simulink model "untitled"  (Simulink 7.9)
settings: Solver=ode45  StartTime=0.0  StopTime=10.0  RelTol=1e-3
settings Model: Creator=Administrator  LastModifiedBy=Administrator

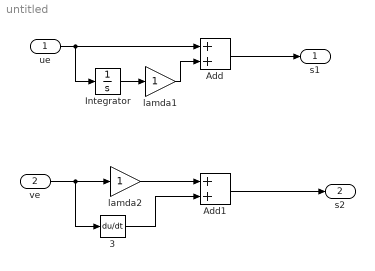
== system untitled ==
  ue : Inport
  ve : Inport  Port=2
  "   3" : Derivative
  Add : Sum
  Add1 : Sum
  Integrator : Integrator
  lamda1 : Gain
  lamda2 : Gain
  s1 : Outport
  s2 : Outport  Port=2
  wires:
  ue/1 -> Add/1, Integrator/1
  Integrator/1 -> lamda1/1
  lamda1/1 -> Add/2
  Add/1 -> s1/1
  ve/1 -> lamda2/1, "   3"/1
  lamda2/1 -> Add1/1
  "   3"/1 -> Add1/2
  Add1/1 -> s2/1
